simulink model "Cardiovascular-Control-System-Simulation"  (R2024b)
settings: Solver=ode5  StartTime=0.0  StopTime=300  FixedStep=0.1  RelTol=1e-3
values from neighbouring files (symbols this model uses):
  Ap = 2.5    [Script_1.m]
  As = 0.1    [Script_1.m]
  fp = 0.2    [Script_1.m]
  fs = 0.015    [Script_1.m]
  Kp = 6    [Script_1.m]
  Ks = 1    [Script_1.m]
libraries: simulink x1, simulink_extras x1
settings Model: Creator=nafis  LastModifiedBy=nafis
settings SolverCC: DateTimeAtSimulationTimeZero=[]

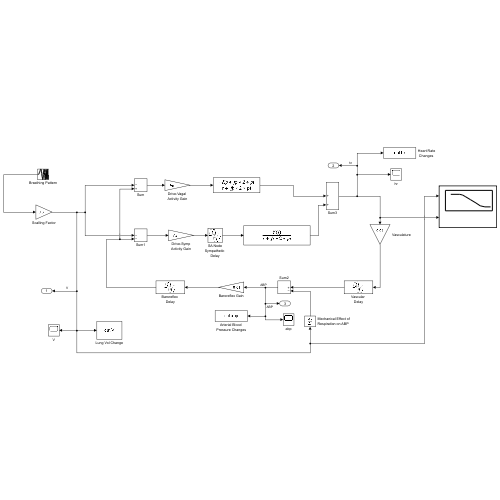
[thumbnail: Simulink's stored preview of the top-level diagram]
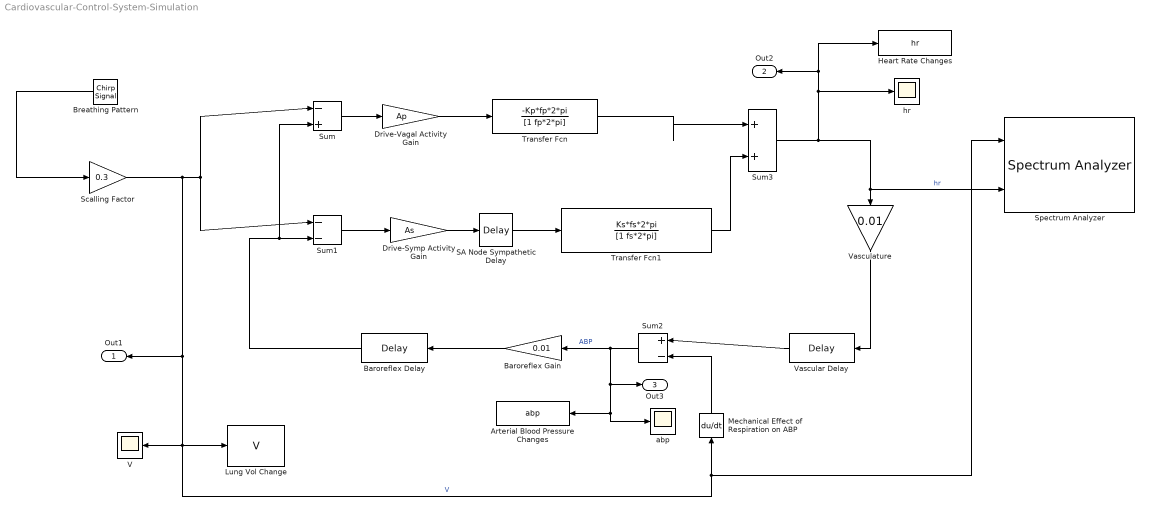
== system Cardiovascular-Control-System-Simulation ==
  Arterial Blood Pressure Changes : ToWorkspace  VariableName=abp  SampleTime=-1
  Baroreflex Delay : TransportDelay  DelayTime=0.3
  Baroreflex Gain : Gain  Gain=0.01
  Breathing Pattern : simulink/Sources/Chirp Signal  f1=0.005  T=300  f2=0.5
  Drive-Symp Activity Gain : Gain  Gain=As
  Drive-Vagal Activity Gain : Gain  Gain=Ap
  Heart Rate Changes : ToWorkspace  VariableName=hr  SampleTime=-1
  Lung Vol Change : ToWorkspace  VariableName=V  SampleTime=-1
  Mechanical Effect of Respiration on ABP : Derivative
  SA Node Sympathetic Delay : TransportDelay  DelayTime=1.7
  Scalling Factor : Gain  Gain=0.3
  Spectrum Analyzer : simulink_extras/Additional Sinks/Spectrum Analyzer  npts=256  fftpts=256  HowOften=64  sampleT=0.1
  Sum : Sum  Inputs=|-+
  Sum1 : Sum  Inputs=|--
  Sum2 : Sum  Inputs=|+-
  Sum3 : Sum  Inputs=|++
  Transfer Fcn : TransferFcn  Numerator=-Kp*fp*2*pi  Denominator=[1 fp*2*pi]
  Transfer Fcn1 : TransferFcn  Numerator=Ks*fs*2*pi  Denominator=[1 fs*2*pi]
  V : Scope
  Vascular Delay : TransportDelay  DelayTime=0.42
  Vasculature : Gain  Gain=0.01
  abp : Scope
  hr : Scope
  Out1 : Outport
  Out2 : Outport  Port=2
  Out3 : Outport  Port=3
  wires:
  Scalling Factor/1 -> Sum1/1, Sum/1, V/1, Lung Vol Change/1, Spectrum Analyzer/1, Mechanical Effect of Respiration on ABP/1, Out1/1  "V"
  Sum1/1 -> Drive-Symp Activity Gain/1
  Sum/1 -> Drive-Vagal Activity Gain/1
  Drive-Vagal Activity Gain/1 -> Transfer Fcn/1
  Transfer Fcn/1 -> Sum3/1
  Transfer Fcn1/1 -> Sum3/2
  Breathing Pattern/1 -> Scalling Factor/1
  Drive-Symp Activity Gain/1 -> SA Node Sympathetic Delay/1
  SA Node Sympathetic Delay/1 -> Transfer Fcn1/1
  Baroreflex Gain/1 -> Baroreflex Delay/1
  Baroreflex Delay/1 -> Sum1/2, Sum/2
  Sum2/1 -> Out3/1, abp/1, Arterial Blood Pressure Changes/1, Baroreflex Gain/1  "ABP"
  Vasculature/1 -> Vascular Delay/1
  Vascular Delay/1 -> Sum2/1
  Sum3/1 -> Heart Rate Changes/1, Out2/1, hr/1, Spectrum Analyzer/2, Vasculature/1  "hr"
  Mechanical Effect of Respiration on ABP/1 -> Sum2/2
